simulink model "LVD_Data_ETR07"  (R2017b)
settings: Solver=FixedStepAuto  StartTime=0.0  StopTime=10.0  RelTol=1e-3
settings Model: Creator=cspt  LastModifiedBy=cspt
settings RTWCC: SystemTargetFile=irt.tlc  TemplateMakefile=irt_default_tmf  Description=INTECRIO Real-Time Target
settings STFCustomTargetCC: TargetLangStandard=C99 (ISO)  UtilityFuncGeneration=Shared location  SystemTargetFile=irt.tlc
settings GRTTargetCC: UtilityFuncGeneration=Shared location  ParMdlRefBuildCompliant=off  CompOptLevelCompliant=off  ConcurrentExecutionCompliant=off  CombineOutputUpdateFcns=off  MatFileLogging=off  CPPClassGenCompliant=off  GRTInterface=on  UseToolchainInfoCompliant=off  GenerateASAP2=on

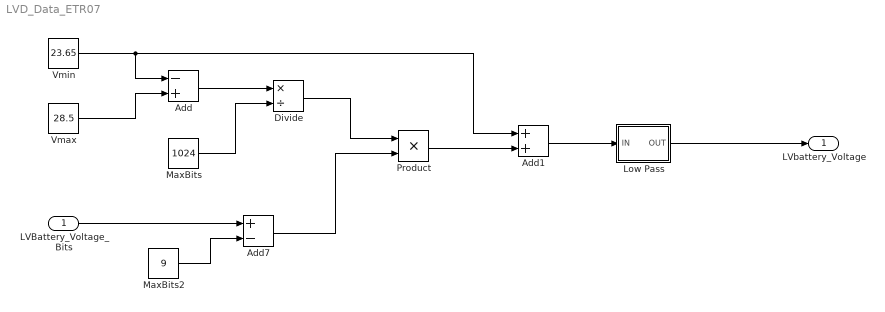
== system LVD_Data_ETR07 ==
  LVBattery_Voltage_Bits : Inport
  Add : Sum  Inputs=-+
  Add1 : Sum
  Add7 : Sum  Inputs=+-
  Divide : Product  Inputs=*/
  Low Pass : Subsystem  TreatAsAtomicUnit=on
  MaxBits : Constant  Value=1024
  MaxBits2 : Constant  Value=9
  Product : Product
  Vmax : Constant  Value=28.5
  Vmin : Constant  Value=23.65
  LVbattery_Voltage : Outport
  wires:
  MaxBits2/1 -> Add7/2
  Low Pass/1(OUT) -> LVbattery_Voltage/1
  Vmin/1 -> Add1/1, Add/1
  LVBattery_Voltage_Bits/1 -> Add7/1
  MaxBits/1 -> Divide/2
  Product/1 -> Add1/2
  Add7/1 -> Product/2
  Add/1 -> Divide/1
  Vmax/1 -> Add/2
  Divide/1 -> Product/1
  Add1/1 -> Low Pass/1(IN)

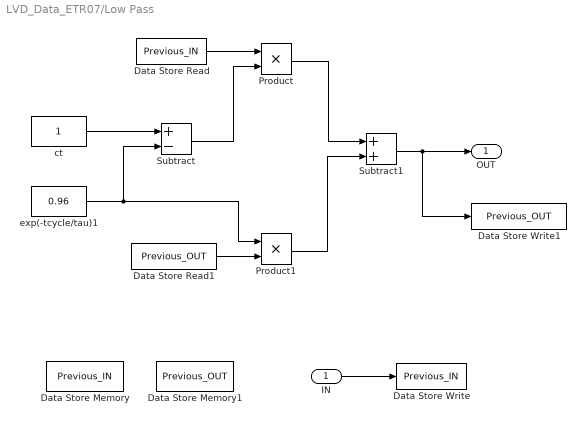
== system LVD_Data_ETR07/Low Pass ==
  IN : Inport
  Data Store Memory : DataStoreMemory  DataStoreName=Previous_IN  ReadBeforeWriteMsg=warning  WriteAfterWriteMsg=warning  WriteAfterReadMsg=warning  ShowAdditionalParam=off
  Data Store Memory1 : DataStoreMemory  DataStoreName=Previous_OUT  ReadBeforeWriteMsg=warning  WriteAfterWriteMsg=warning  WriteAfterReadMsg=warning  ShowAdditionalParam=off
  Data Store Read : DataStoreRead  DataStoreName=Previous_IN
  Data Store Read1 : DataStoreRead  DataStoreName=Previous_OUT
  Data Store Write : DataStoreWrite  DataStoreName=Previous_IN
  Data Store Write1 : DataStoreWrite  DataStoreName=Previous_OUT
  Product : Product
  Product1 : Product
  Subtract : Sum  Inputs=+-
  Subtract1 : Sum
  ct : Constant
  exp(-tcycle/tau)1 : Constant  Value=0.96
  OUT : Outport
  wires:
  IN/1 -> Data Store Write/1
  Data Store Read/1 -> Product/1
  Data Store Read1/1 -> Product1/2
  ct/1 -> Subtract/1
  Subtract/1 -> Product/2
  exp(-tcycle/tau)1/1 -> Product1/1, Subtract/2
  Product/1 -> Subtract1/1
  Product1/1 -> Subtract1/2
  Subtract1/1 -> Data Store Write1/1, OUT/1
